simulink model "CruiseControllerSimR2017a"  (R2017a)
settings: Solver=VariableStepAuto  StartTime=0.0  StopTime=10.0  RelTol=1e-3
values from neighbouring files (symbols this model uses):
  EndVel = (Time2-Time1)*Slope+StartVel    (= 31.525)    [CruiseControllerSimScript.m]
  InputNum = 3    [CruiseControllerSimScript.m]
  InputTime = 0    [CruiseControllerSimScript.m]
  Ki = 1    [CruiseControllerSimScript.m]
  Kp = 1    [CruiseControllerSimScript.m]
  Slope = 0.5*g    (= 4.905)    [CruiseControllerSimScript.m]
  StartVel = 7    [CruiseControllerSimScript.m]
  tau = .5    (= 0.5)    [CruiseControllerSimScript.m]
  Time1 = 2    [CruiseControllerSimScript.m]
  Time2 = Time1 + DTime    (= 7)    [CruiseControllerSimScript.m]
undefined symbols (not defined in the file or in its folder): heaviside
libraries: simulink x2
settings Model: Creator=domin  LastModifiedBy=domin

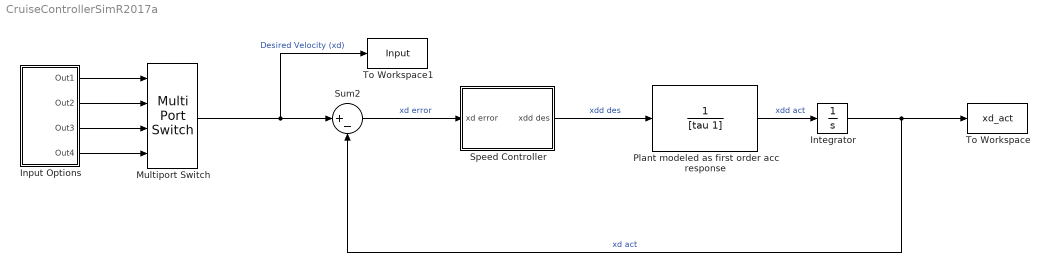
== system CruiseControllerSimR2017a ==
  Input Options : Subsystem
  Integrator : Integrator
  Multiport Switch : MultiPortSwitch
  Plant modeled as first order acc response : TransferFcn  Denominator=[tau 1]
  Speed Controller : Subsystem
  Sum2 : Sum  Inputs=|+-
  To Workspace : ToWorkspace  VariableName=xd_act  SampleTime=-1
  To Workspace1 : ToWorkspace  VariableName=Input  SampleTime=-1
  wires:
  Multiport Switch/1 -> To Workspace1/1, Sum2/1  "Desired Velocity (xd)"
  Input Options/2(Out2) -> Multiport Switch/2
  Speed Controller/1(xdd des) -> Plant modeled as first order acc response/1  "xdd des"
  Input Options/4(Out4) -> Multiport Switch/4
  Input Options/3(Out3) -> Multiport Switch/3
  Integrator/1 -> Sum2/2, To Workspace/1  "xd act"
  Sum2/1 -> Speed Controller/1(xd error)  "xd error"
  Plant modeled as first order acc response/1 -> Integrator/1  "xdd act"
  Input Options/1(Out1) -> Multiport Switch/1

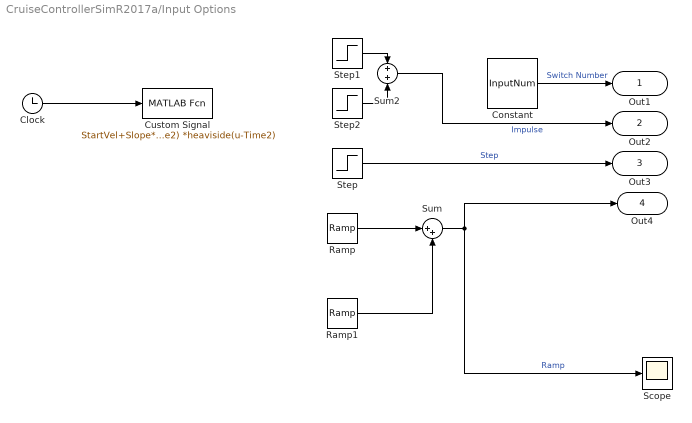
== system CruiseControllerSimR2017a/Input Options ==
  Clock : Clock
  Constant : Constant  Value=InputNum
  Custom Signal : MATLABFcn  MATLABFcn=StartVel+Slope*(u-Time1) *heaviside(u-Time1)-Slope*(u-Time2) *heaviside(u-Time2)  OutputDimensions=1
  Ramp : simulink/Sources/Ramp  slope=Slope  start=Time1  X0=StartVel
  Ramp1 : simulink/Sources/Ramp  slope=-Slope  start=Time2  X0=0
  Scope : Scope
  Step : Step  Time=InputTime  Before=StartVel  After=EndVel  SampleTime=0
  Step1 : Step  Time=InputTime  Before=StartVel  After=StartVel+(1*10^10)  SampleTime=0
  Step2 : Step  Time=InputTime + (1*10^-10)  After=-(1*10^10)  SampleTime=0
  Sum : Sum  Inputs=|++
  Sum2 : Sum
  Out1 : Outport
  Out2 : Outport  Port=2
  Out3 : Outport  Port=3
  Out4 : Outport  Port=4
  wires:
  Clock/1 -> Custom Signal/1
  Sum2/1 -> Out2/1  "Impulse"
  Constant/1 -> Out1/1  "Switch Number"
  Step2/1 -> Sum2/2
  Step1/1 -> Sum2/1
  Step/1 -> Out3/1  "Step"
  Ramp/1 -> Sum/1
  Ramp1/1 -> Sum/2
  Sum/1 -> Out4/1, Scope/1  "Ramp"

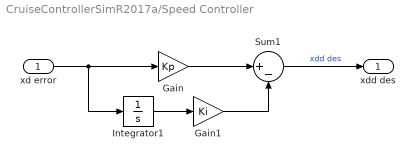
== system CruiseControllerSimR2017a/Speed Controller ==
  xd error : Inport
  Gain : Gain  Gain=Kp
  Gain1 : Gain  Gain=Ki
  Integrator1 : Integrator
  Sum1 : Sum  Inputs=|+-
  xdd des : Outport
  wires:
  xd error/1 -> Gain/1, Integrator1/1
  Integrator1/1 -> Gain1/1
  Gain1/1 -> Sum1/2
  Sum1/1 -> xdd des/1  "xdd des"
  Gain/1 -> Sum1/1
